simulink model "cpu_von_nuemann"  (R2020a)
settings: Solver=VariableStepAuto  StartTime=0.0  StopTime=10.0  RelTol=1e-3
libraries: simulink_extras x402, msbPllFoundation x1
(part 3 of 64)

== system cpu_von_nuemann/CPU/ALU/Multiplier/Subsystem3 ==
  In1 : Inport
  In2 : Inport  Port=2
  Constant17 : Constant  Value=0
  Demux : Demux  Outputs=16
  Demux1 : Demux  Outputs=16
  Display1 : Display
  Logical Operator : Logic  Operator=XOR  AllPortsSameDT=off  OutDataTypeStr=boolean
  Logical Operator1 : Logic  AllPortsSameDT=off  OutDataTypeStr=boolean
  Mux : Mux  Inputs=16
  Mux1 : Mux  Inputs=16
  Subsystem : Subsystem
  Subsystem1 : Subsystem
  Subsystem2 : Subsystem
  Subsystem3 : Subsystem
  Subsystem4 : Subsystem
  Subsystem5 : Subsystem
  Subsystem6 : Subsystem
  Out1 : Outport
  Out2 : Outport  Port=2
  wires:
  Subsystem3/11(Out11) -> Subsystem/27(In27)
  Subsystem5/16(Out16) -> Mux1/7
  Subsystem/16(Out16) -> Subsystem5/15(In23)
  Subsystem5/7(Out7) -> Subsystem6/30(In30)
  Subsystem2/14(Out14) -> Subsystem/14(In22)
  Subsystem4/9(Out9) -> Mux1/9
  Subsystem5/11(Out11) -> Mux1/2
  Subsystem2/15(Out15) -> Subsystem/15(In23)
  Subsystem3/16(Out16) -> Subsystem/32(In32)
  Subsystem3/6(Out6) -> Subsystem/22(In14)
  Subsystem6/10(Out10) -> Mux/9
  Subsystem5/2(Out2) -> Subsystem6/25(In25)
  Subsystem4/7(Out7) -> Subsystem5/31(In31)
  Subsystem2/11(Out11) -> Subsystem/11(In19)
  Subsystem3/9(Out9) -> Subsystem/25(In25)
  Subsystem1/2(Out2) -> Subsystem6/2(In2)
  Subsystem1/3(Out3) -> Subsystem6/3(In3)
  Subsystem/17(Out17) -> Subsystem5/16(In24)
  Subsystem/4(Out4) -> Subsystem5/3(In3)
  Subsystem3/8(Out8) -> Subsystem/24(In16)
  Subsystem/11(Out11) -> Subsystem5/10(In18)
  Logical Operator1/1 -> Subsystem6/23(In15)
  Subsystem3/2(Out2) -> Subsystem/18(In10)
  Subsystem1/13(Out13) -> Subsystem6/13(14)
  Subsystem4/4(Out4) -> Subsystem5/28(In28)
  Subsystem5/17(Out17) -> Mux1/8
  Subsystem5/5(Out5) -> Subsystem6/28(In28)
  Subsystem1/8(Out8) -> Subsystem6/8(In8)
  Subsystem2/3(Out3) -> Subsystem/3(In3)
  Subsystem5/6(Out6) -> Subsystem6/29(In29)
  Subsystem/2(Out2) -> Subsystem5/1(In1)
  Subsystem4/1(Out1) -> Subsystem5/25(In25)
  Subsystem1/7(Out7) -> Subsystem6/7(In7)
  Subsystem5/9(Out9) -> Subsystem6/32(In32)
  Subsystem6/8(Out8) -> Mux/7
  Subsystem1/5(Out5) -> Subsystem6/5(In5)
  Subsystem6/11(Out11) -> Mux/10
  Subsystem1/6(Out6) -> Subsystem6/6(In6)
  Subsystem/7(Out7) -> Subsystem5/6(In6)
  Subsystem2/16(Out16) -> Subsystem/16(In24)
  Demux/7 -> Subsystem2/7(In7), Subsystem1/7(In7)
  Demux1/14 -> Subsystem4/14(In14), Subsystem2/14(In14)
  Demux/16 -> Subsystem4/8(In8), Subsystem3/8(In8)
  Subsystem2/1(Out1) -> Subsystem/1(In1)
  Subsystem5/15(Out15) -> Mux1/6
  Subsystem4/16(Out16) -> Mux1/16
  Subsystem3/4(Out4) -> Subsystem/20(In12)
  Subsystem/1(Out1) -> Logical Operator1/2, Logical Operator/2
  Subsystem1/4(Out4) -> Subsystem6/4(In4)
  Subsystem4/11(Out11) -> Mux1/11
  Demux/1 -> Subsystem1/1(In1), Subsystem2/1(In1)
  Subsystem3/10(Out10) -> Subsystem/26(In26)
  Subsystem6/2(Out2) -> Mux/1
  Subsystem/9(Out9) -> Subsystem5/8(In8)
  Demux1/3 -> Subsystem3/11(In11), Subsystem1/11(In11)
  Demux1/7 -> Subsystem3/15(In15), Subsystem1/15(In15)
  Subsystem/5(Out5) -> Subsystem5/4(In4)
  Mux/1 -> Out1/1
  Subsystem5/10(Out10) -> Mux1/1
  Subsystem1/12(Out12) -> Subsystem6/12(In20)
  Subsystem2/6(Out6) -> Subsystem/6(In6)
  Demux/13 -> Subsystem4/5(In5), Subsystem3/5(In5)
  Demux/10 -> Subsystem4/2(In2), Subsystem3/2(In2)
  Demux/11 -> Subsystem4/3(In3), Subsystem3/3(In3)
  Subsystem1/11(Out11) -> Subsystem6/11(In19)
  Subsystem6/17(Out17) -> Mux/16
  Demux/9 -> Subsystem4/1(In1), Subsystem3/1(In1)
  Subsystem4/15(Out15) -> Mux1/15
  Subsystem5/8(Out8) -> Subsystem6/31(In31)
  Demux1/1 -> Subsystem1/9(In9), Subsystem3/9(In9)
  Demux1/2 -> Subsystem3/10(In10), Subsystem1/10(In10)
  Demux/8 -> Subsystem2/8(In8), Subsystem1/8(In8)
  Demux/14 -> Subsystem4/6(In6), Subsystem3/6(In6)
  Subsystem1/15(Out15) -> Subsystem6/15(In23)
  Demux1/9 -> Subsystem2/9(In9), Subsystem4/9(In9)
  Subsystem5/14(Out14) -> Mux1/5
  Demux/6 -> Subsystem1/6(In6), Subsystem2/6(In6)
  Subsystem2/7(Out7) -> Subsystem/7(In7)
  Subsystem2/4(Out4) -> Subsystem/4(In4)
  Demux1/5 -> Subsystem3/13(In13), Subsystem1/13(In13)
  Subsystem/8(Out8) -> Subsystem5/7(In7)
  Logical Operator/1 -> Subsystem6/24(In16)
  Demux1/12 -> Subsystem2/12(In12), Subsystem4/12(In12)
  Subsystem2/9(Out9) -> Subsystem/9(In17)
  Subsystem5/13(Out13) -> Mux1/4
  Subsystem5/3(Out3) -> Subsystem6/26(In26)
  Demux1/8 -> Subsystem1/16(In16), Subsystem3/16(In16)
  Subsystem4/14(Out14) -> Mux1/14
  Constant17/1 -> Subsystem5/24(In16), Subsystem5/23(In15), Subsystem5/22(In14), Subsystem5/21(In13), Subsystem5/20(In12), Subsystem5/19(In11), Subsystem5/18(In10), Subsystem5/17(In9), Subsystem6/17(In9), Subsystem6/18(In10), Subsystem6/20(In12), Subsystem6/21(In13), Subsystem6/22(In14), Subsystem6/19(In11)
  Subsystem3/13(Out13) -> Subsystem/29(In29)
  Subsystem1/16(Out16) -> Subsystem6/16(In24)
  Subsystem/15(Out15) -> Subsystem5/14(In22)
  Demux1/13 -> Subsystem2/13(In13), Subsystem4/13(In13)
  Subsystem/12(Out12) -> Subsystem5/11(In19)
  Demux1/16 -> Subsystem2/16(In16), Subsystem4/16(In16)
  Subsystem5/12(Out12) -> Mux1/3
  Subsystem3/15(Out15) -> Subsystem/31(In31)
  Subsystem6/9(Out9) -> Mux/8
  Demux/5 -> Subsystem1/5(In5), Subsystem2/5(In5)
  Subsystem6/4(Out4) -> Mux/3
  Subsystem6/3(Out3) -> Mux/2
  Subsystem4/13(Out13) -> Mux1/13
  Demux1/6 -> Subsystem3/14(In14), Subsystem1/14(In14)
  Subsystem/6(Out6) -> Subsystem5/5(In5)
  Subsystem/13(Out13) -> Subsystem5/12(In20)
  Subsystem6/13(Out13) -> Mux/12
  Subsystem6/12(Out12) -> Mux/11
  Subsystem4/10(Out10) -> Mux1/10
  Subsystem3/5(Out5) -> Subsystem/21(In13)
  Subsystem/10(Out10) -> Subsystem5/9(In17)
  Subsystem2/12(Out12) -> Subsystem/12(In20)
  Subsystem5/1(Out1) -> Logical Operator/1, Logical Operator1/1
  Subsystem6/5(Out5) -> Mux/4
  Subsystem3/1(Out1) -> Subsystem/17(In9)
  Subsystem4/8(Out8) -> Subsystem5/32(In32)
  Subsystem3/12(Out12) -> Subsystem/28(In28)
  Subsystem6/1(Out1) -> Display1/1
  Subsystem4/6(Out6) -> Subsystem5/30(In30)
  Subsystem2/2(Out2) -> Subsystem/2(In2)
  Subsystem2/10(Out10) -> Subsystem/10(In18)
  Subsystem4/5(Out5) -> Subsystem5/29(In29)
  Subsystem2/13(Out13) -> Subsystem/13(14)
  Subsystem1/1(Out1) -> Subsystem6/1(In1)
  Subsystem6/7(Out7) -> Mux/6
  Subsystem6/14(Out14) -> Mux/13
  Subsystem5/4(Out4) -> Subsystem6/27(In27)
  Subsystem2/8(Out8) -> Subsystem/8(In8)
  Subsystem/14(Out14) -> Subsystem5/13(14)
  Subsystem6/16(Out16) -> Mux/15
  Demux/4 -> Subsystem2/4(In4), Subsystem1/4(In4)
  Subsystem1/10(Out10) -> Subsystem6/10(In18)
  Demux/12 -> Subsystem4/4(In4), Subsystem3/4(In4)
  Subsystem3/14(Out14) -> Subsystem/30(In30)
  Subsystem2/5(Out5) -> Subsystem/5(In5)
  Demux1/10 -> Subsystem2/10(In10), Subsystem4/10(In10)
  Demux/2 -> Subsystem1/2(In2), Subsystem2/2(In2)
  Subsystem6/6(Out6) -> Mux/5
  Subsystem/3(Out3) -> Subsystem5/2(In2)
  Subsystem4/12(Out12) -> Mux1/12
  Demux1/4 -> Subsystem1/12(In12), Subsystem3/12(In12)
  Demux/15 -> Subsystem4/7(In7), Subsystem3/7(In7)
  Subsystem1/14(Out14) -> Subsystem6/14(In22)
  Subsystem3/3(Out3) -> Subsystem/19(In11)
  Subsystem6/15(Out15) -> Mux/14
  Subsystem1/9(Out9) -> Subsystem6/9(In17)
  Demux1/11 -> Subsystem2/11(In11), Subsystem4/11(In11)
  Subsystem4/2(Out2) -> Subsystem5/26(In26)
  Demux/3 -> Subsystem1/3(In3), Subsystem2/3(In3)
  Subsystem4/3(Out3) -> Subsystem5/27(In27)
  Subsystem3/7(Out7) -> Subsystem/23(In15)
  Demux1/15 -> Subsystem2/15(In15), Subsystem4/15(In15)
  In1/1 -> Demux/1
  In2/1 -> Demux1/1
  Mux1/1 -> Out2/1

== system cpu_von_nuemann/CPU/ALU/Multiplier/Subsystem4 ==
  In1 : Inport
  In2 : Inport  Port=2
  In3 : Inport  Port=3
  Demux : Demux  Outputs=2
  Demux1 : Demux  Outputs=2
  Mux : Mux  Inputs=2
  Subsystem1 : Subsystem
  Subsystem2 : Subsystem
  Out1 : Outport
  Out2 : Outport  Port=2
  wires:
  Mux/1 -> Out2/1
  In3/1 -> Demux1/1
  Subsystem2/2(Out2) -> Mux/2
  In1/1 -> Demux/1
  Subsystem2/1(Out1) -> Subsystem1/2(In2)
  Subsystem1/2(Out2) -> Mux/1
  Demux1/2 -> Subsystem2/3(In3)
  In2/1 -> Subsystem2/2(In2)
  Demux/2 -> Subsystem2/1(In1)
  Subsystem1/1(Out1) -> Out1/1
  Demux1/1 -> Subsystem1/3(In3)
  Demux/1 -> Subsystem1/1(In1)

== system cpu_von_nuemann/CPU/ALU/Multiplier/Subsystem5 ==
  In1 : Inport
  In2 : Inport  Port=2
  In3 : Inport  Port=3
  Demux : Demux  Outputs=2
  Demux1 : Demux  Outputs=2
  Mux : Mux  Inputs=2
  Subsystem : Subsystem
  Subsystem1 : Subsystem
  Out1 : Outport
  Out2 : Outport  Port=2
  wires:
  Mux/1 -> Out2/1
  Subsystem1/2(Out2) -> Mux/1
  In2/1 -> Subsystem/2(In2)
  Subsystem1/1(Out1) -> Out1/1
  Demux/2 -> Subsystem/1(In1)
  In3/1 -> Demux1/1
  Demux1/2 -> Subsystem/3(In3)
  Demux/1 -> Subsystem1/1(In1)
  Demux1/1 -> Subsystem1/3(In3)
  In1/1 -> Demux/1
  Subsystem/2(Out2) -> Mux/2
  Subsystem/1(Out1) -> Subsystem1/2(In2)

== system cpu_von_nuemann/CPU/ALU/Multiplier/Subsystem7 ==
  In1 : Inport
  In2 : Inport  Port=2
  Constant17 : Constant  Value=0
  Demux : Demux  Outputs=16
  Demux1 : Demux  Outputs=16
  Display1 : Display
  Logical Operator : Logic  Operator=XOR  AllPortsSameDT=off  OutDataTypeStr=boolean
  Logical Operator1 : Logic  AllPortsSameDT=off  OutDataTypeStr=boolean
  Mux : Mux  Inputs=16
  Mux1 : Mux  Inputs=16
  Subsystem : Subsystem
  Subsystem1 : Subsystem
  Subsystem2 : Subsystem
  Subsystem3 : Subsystem
  Subsystem4 : Subsystem
  Subsystem5 : Subsystem
  Subsystem6 : Subsystem
  Out1 : Outport
  Out2 : Outport  Port=2
  wires:
  Subsystem3/11(Out11) -> Subsystem/27(In27)
  Subsystem5/16(Out16) -> Mux1/7
  Subsystem/16(Out16) -> Subsystem5/15(In23)
  Subsystem5/7(Out7) -> Subsystem6/30(In30)
  Subsystem2/14(Out14) -> Subsystem/14(In22)
  Subsystem4/9(Out9) -> Mux1/9
  Subsystem5/11(Out11) -> Mux1/2
  Subsystem2/15(Out15) -> Subsystem/15(In23)
  Subsystem3/16(Out16) -> Subsystem/32(In32)
  Subsystem3/6(Out6) -> Subsystem/22(In14)
  Subsystem6/10(Out10) -> Mux/9
  Subsystem5/2(Out2) -> Subsystem6/25(In25)
  Subsystem4/7(Out7) -> Subsystem5/31(In31)
  Subsystem2/11(Out11) -> Subsystem/11(In19)
  Subsystem3/9(Out9) -> Subsystem/25(In25)
  Subsystem1/2(Out2) -> Subsystem6/2(In2)
  Subsystem1/3(Out3) -> Subsystem6/3(In3)
  Subsystem/17(Out17) -> Subsystem5/16(In24)
  Subsystem/4(Out4) -> Subsystem5/3(In3)
  Subsystem3/8(Out8) -> Subsystem/24(In16)
  Subsystem/11(Out11) -> Subsystem5/10(In18)
  Logical Operator1/1 -> Subsystem6/23(In15)
  Subsystem3/2(Out2) -> Subsystem/18(In10)
  Subsystem1/13(Out13) -> Subsystem6/13(14)
  Subsystem4/4(Out4) -> Subsystem5/28(In28)
  Subsystem5/17(Out17) -> Mux1/8
  Subsystem5/5(Out5) -> Subsystem6/28(In28)
  Subsystem1/8(Out8) -> Subsystem6/8(In8)
  Subsystem2/3(Out3) -> Subsystem/3(In3)
  Subsystem5/6(Out6) -> Subsystem6/29(In29)
  Subsystem/2(Out2) -> Subsystem5/1(In1)
  Subsystem4/1(Out1) -> Subsystem5/25(In25)
  Subsystem1/7(Out7) -> Subsystem6/7(In7)
  Subsystem5/9(Out9) -> Subsystem6/32(In32)
  Subsystem6/8(Out8) -> Mux/7
  Subsystem1/5(Out5) -> Subsystem6/5(In5)
  Subsystem6/11(Out11) -> Mux/10
  Subsystem1/6(Out6) -> Subsystem6/6(In6)
  Subsystem/7(Out7) -> Subsystem5/6(In6)
  Subsystem2/16(Out16) -> Subsystem/16(In24)
  Demux/7 -> Subsystem2/7(In7), Subsystem1/7(In7)
  Demux1/14 -> Subsystem4/14(In14), Subsystem2/14(In14)
  Demux/16 -> Subsystem4/8(In8), Subsystem3/8(In8)
  Subsystem2/1(Out1) -> Subsystem/1(In1)
  Subsystem5/15(Out15) -> Mux1/6
  Subsystem4/16(Out16) -> Mux1/16
  Subsystem3/4(Out4) -> Subsystem/20(In12)
  Subsystem/1(Out1) -> Logical Operator1/2, Logical Operator/2
  Subsystem1/4(Out4) -> Subsystem6/4(In4)
  Subsystem4/11(Out11) -> Mux1/11
  Demux/1 -> Subsystem1/1(In1), Subsystem2/1(In1)
  Subsystem3/10(Out10) -> Subsystem/26(In26)
  Subsystem6/2(Out2) -> Mux/1
  Subsystem/9(Out9) -> Subsystem5/8(In8)
  Demux1/3 -> Subsystem3/11(In11), Subsystem1/11(In11)
  Demux1/7 -> Subsystem3/15(In15), Subsystem1/15(In15)
  Subsystem/5(Out5) -> Subsystem5/4(In4)
  Mux/1 -> Out1/1
  Subsystem5/10(Out10) -> Mux1/1
  Subsystem1/12(Out12) -> Subsystem6/12(In20)
  Subsystem2/6(Out6) -> Subsystem/6(In6)
  Demux/13 -> Subsystem4/5(In5), Subsystem3/5(In5)
  Demux/10 -> Subsystem4/2(In2), Subsystem3/2(In2)
  Demux/11 -> Subsystem4/3(In3), Subsystem3/3(In3)
  Subsystem1/11(Out11) -> Subsystem6/11(In19)
  Subsystem6/17(Out17) -> Mux/16
  Demux/9 -> Subsystem4/1(In1), Subsystem3/1(In1)
  Subsystem4/15(Out15) -> Mux1/15
  Subsystem5/8(Out8) -> Subsystem6/31(In31)
  Demux1/1 -> Subsystem1/9(In9), Subsystem3/9(In9)
  Demux1/2 -> Subsystem3/10(In10), Subsystem1/10(In10)
  Demux/8 -> Subsystem2/8(In8), Subsystem1/8(In8)
  Demux/14 -> Subsystem4/6(In6), Subsystem3/6(In6)
  Subsystem1/15(Out15) -> Subsystem6/15(In23)
  Demux1/9 -> Subsystem2/9(In9), Subsystem4/9(In9)
  Subsystem5/14(Out14) -> Mux1/5
  Demux/6 -> Subsystem1/6(In6), Subsystem2/6(In6)
  Subsystem2/7(Out7) -> Subsystem/7(In7)
  Subsystem2/4(Out4) -> Subsystem/4(In4)
  Demux1/5 -> Subsystem3/13(In13), Subsystem1/13(In13)
  Subsystem/8(Out8) -> Subsystem5/7(In7)
  Logical Operator/1 -> Subsystem6/24(In16)
  Demux1/12 -> Subsystem2/12(In12), Subsystem4/12(In12)
  Subsystem2/9(Out9) -> Subsystem/9(In17)
  Subsystem5/13(Out13) -> Mux1/4
  Subsystem5/3(Out3) -> Subsystem6/26(In26)
  Demux1/8 -> Subsystem1/16(In16), Subsystem3/16(In16)
  Subsystem4/14(Out14) -> Mux1/14
  Constant17/1 -> Subsystem5/24(In16), Subsystem5/23(In15), Subsystem5/22(In14), Subsystem5/21(In13), Subsystem5/20(In12), Subsystem5/19(In11), Subsystem5/18(In10), Subsystem5/17(In9), Subsystem6/17(In9), Subsystem6/18(In10), Subsystem6/20(In12), Subsystem6/21(In13), Subsystem6/22(In14), Subsystem6/19(In11)
  Subsystem3/13(Out13) -> Subsystem/29(In29)
  Subsystem1/16(Out16) -> Subsystem6/16(In24)
  Subsystem/15(Out15) -> Subsystem5/14(In22)
  Demux1/13 -> Subsystem2/13(In13), Subsystem4/13(In13)
  Subsystem/12(Out12) -> Subsystem5/11(In19)
  Demux1/16 -> Subsystem2/16(In16), Subsystem4/16(In16)
  Subsystem5/12(Out12) -> Mux1/3
  Subsystem3/15(Out15) -> Subsystem/31(In31)
  Subsystem6/9(Out9) -> Mux/8
  Demux/5 -> Subsystem1/5(In5), Subsystem2/5(In5)
  Subsystem6/4(Out4) -> Mux/3
  Subsystem6/3(Out3) -> Mux/2
  Subsystem4/13(Out13) -> Mux1/13
  Demux1/6 -> Subsystem3/14(In14), Subsystem1/14(In14)
  Subsystem/6(Out6) -> Subsystem5/5(In5)
  Subsystem/13(Out13) -> Subsystem5/12(In20)
  Subsystem6/13(Out13) -> Mux/12
  Subsystem6/12(Out12) -> Mux/11
  Subsystem4/10(Out10) -> Mux1/10
  Subsystem3/5(Out5) -> Subsystem/21(In13)
  Subsystem/10(Out10) -> Subsystem5/9(In17)
  Subsystem2/12(Out12) -> Subsystem/12(In20)
  Subsystem5/1(Out1) -> Logical Operator/1, Logical Operator1/1
  Subsystem6/5(Out5) -> Mux/4
  Subsystem3/1(Out1) -> Subsystem/17(In9)
  Subsystem4/8(Out8) -> Subsystem5/32(In32)
  Subsystem3/12(Out12) -> Subsystem/28(In28)
  Subsystem6/1(Out1) -> Display1/1
  Subsystem4/6(Out6) -> Subsystem5/30(In30)
  Subsystem2/2(Out2) -> Subsystem/2(In2)
  Subsystem2/10(Out10) -> Subsystem/10(In18)
  Subsystem4/5(Out5) -> Subsystem5/29(In29)
  Subsystem2/13(Out13) -> Subsystem/13(14)
  Subsystem1/1(Out1) -> Subsystem6/1(In1)
  Subsystem6/7(Out7) -> Mux/6
  Subsystem6/14(Out14) -> Mux/13
  Subsystem5/4(Out4) -> Subsystem6/27(In27)
  Subsystem2/8(Out8) -> Subsystem/8(In8)
  Subsystem/14(Out14) -> Subsystem5/13(14)
  Subsystem6/16(Out16) -> Mux/15
  Demux/4 -> Subsystem2/4(In4), Subsystem1/4(In4)
  Subsystem1/10(Out10) -> Subsystem6/10(In18)
  Demux/12 -> Subsystem4/4(In4), Subsystem3/4(In4)
  Subsystem3/14(Out14) -> Subsystem/30(In30)
  Subsystem2/5(Out5) -> Subsystem/5(In5)
  Demux1/10 -> Subsystem2/10(In10), Subsystem4/10(In10)
  Demux/2 -> Subsystem1/2(In2), Subsystem2/2(In2)
  Subsystem6/6(Out6) -> Mux/5
  Subsystem/3(Out3) -> Subsystem5/2(In2)
  Subsystem4/12(Out12) -> Mux1/12
  Demux1/4 -> Subsystem1/12(In12), Subsystem3/12(In12)
  Demux/15 -> Subsystem4/7(In7), Subsystem3/7(In7)
  Subsystem1/14(Out14) -> Subsystem6/14(In22)
  Subsystem3/3(Out3) -> Subsystem/19(In11)
  Subsystem6/15(Out15) -> Mux/14
  Subsystem1/9(Out9) -> Subsystem6/9(In17)
  Demux1/11 -> Subsystem2/11(In11), Subsystem4/11(In11)
  Subsystem4/2(Out2) -> Subsystem5/26(In26)
  Demux/3 -> Subsystem1/3(In3), Subsystem2/3(In3)
  Subsystem4/3(Out3) -> Subsystem5/27(In27)
  Subsystem3/7(Out7) -> Subsystem/23(In15)
  Demux1/15 -> Subsystem2/15(In15), Subsystem4/15(In15)
  In1/1 -> Demux/1
  In2/1 -> Demux1/1
  Mux1/1 -> Out2/1

== system cpu_von_nuemann/CPU/ALU/Subsystem7/Subsystem1 ==
  In20 : Inport
  In21 : Inport  Port=2
  In1 : Inport  Port=3
  In2 : Inport  Port=4
  In3 : Inport  Port=5
  In4 : Inport  Port=6
  In5 : Inport  Port=7
  In6 : Inport  Port=8
  In7 : Inport  Port=9
  In8 : Inport  Port=10
  In9 : Inport  Port=11
  In10 : Inport  Port=12
  In11 : Inport  Port=13
  In12 : Inport  Port=14
  In13 : Inport  Port=15
  In14 : Inport  Port=16
  In15 : Inport  Port=17
  In16 : Inport  Port=18
  In17 : Inport  Port=19
  In18 : Inport  Port=20
  In19 : Inport  Port=21
  Subsystem1 : Subsystem
  Subsystem2 : Subsystem
  Subsystem3 : Subsystem
  Subsystem4 : Subsystem
  Subsystem5 : Subsystem
  Out1 : Outport
  wires:
  Subsystem4/1(Out1) -> Subsystem5/3(In3)
  Subsystem1/1(Out1) -> Subsystem5/4(In4)
  Subsystem2/1(Out1) -> Subsystem5/5(In5)
  Subsystem3/1(Out1) -> Subsystem5/6(In7)
  Subsystem5/1(Out1) -> Out1/1
  In1/1 -> Subsystem4/1(In1), Subsystem1/1(In1), Subsystem3/1(In1), Subsystem2/1(In1)
  In2/1 -> Subsystem4/2(In2), Subsystem1/2(In2), Subsystem3/2(In2), Subsystem2/2(In2)
  In19/1 -> Subsystem5/7(In6), Subsystem3/7(In6), Subsystem2/7(In6), Subsystem1/7(In6), Subsystem4/7(In6)
  In3/1 -> Subsystem4/3(In3)
  In4/1 -> Subsystem4/4(In4)
  In6/1 -> Subsystem4/6(In7)
  In5/1 -> Subsystem4/5(In5)
  In8/1 -> Subsystem1/4(In4)
  In9/1 -> Subsystem1/5(In5)
  In7/1 -> Subsystem1/3(In3)
  In10/1 -> Subsystem1/6(In7)
  In15/1 -> Subsystem3/3(In3)
  In18/1 -> Subsystem3/6(In7)
  In13/1 -> Subsystem2/5(In5)
  In12/1 -> Subsystem2/4(In4)
  In17/1 -> Subsystem3/5(In5)
  In16/1 -> Subsystem3/4(In4)
  In11/1 -> Subsystem2/3(In3)
  In14/1 -> Subsystem2/6(In7)
  In20/1 -> Subsystem5/1(In1)
  In21/1 -> Subsystem5/2(In2)

== system cpu_von_nuemann/CPU/ALU/Subsystem7/Subsystem2 ==
  In20 : Inport
  In21 : Inport  Port=2
  In1 : Inport  Port=3
  In2 : Inport  Port=4
  In3 : Inport  Port=5
  In4 : Inport  Port=6
  In5 : Inport  Port=7
  In6 : Inport  Port=8
  In7 : Inport  Port=9
  In8 : Inport  Port=10
  In9 : Inport  Port=11
  In10 : Inport  Port=12
  In11 : Inport  Port=13
  In12 : Inport  Port=14
  In13 : Inport  Port=15
  In14 : Inport  Port=16
  In15 : Inport  Port=17
  In16 : Inport  Port=18
  In17 : Inport  Port=19
  In18 : Inport  Port=20
  In19 : Inport  Port=21
  Subsystem1 : Subsystem
  Subsystem2 : Subsystem
  Subsystem3 : Subsystem
  Subsystem4 : Subsystem
  Subsystem5 : Subsystem
  Out1 : Outport
  wires:
  Subsystem4/1(Out1) -> Subsystem5/3(In3)
  Subsystem1/1(Out1) -> Subsystem5/4(In4)
  Subsystem2/1(Out1) -> Subsystem5/5(In5)
  Subsystem3/1(Out1) -> Subsystem5/6(In7)
  Subsystem5/1(Out1) -> Out1/1
  In1/1 -> Subsystem4/1(In1), Subsystem1/1(In1), Subsystem3/1(In1), Subsystem2/1(In1)
  In2/1 -> Subsystem4/2(In2), Subsystem1/2(In2), Subsystem3/2(In2), Subsystem2/2(In2)
  In19/1 -> Subsystem5/7(In6), Subsystem3/7(In6), Subsystem2/7(In6), Subsystem1/7(In6), Subsystem4/7(In6)
  In3/1 -> Subsystem4/3(In3)
  In4/1 -> Subsystem4/4(In4)
  In6/1 -> Subsystem4/6(In7)
  In5/1 -> Subsystem4/5(In5)
  In8/1 -> Subsystem1/4(In4)
  In9/1 -> Subsystem1/5(In5)
  In7/1 -> Subsystem1/3(In3)
  In10/1 -> Subsystem1/6(In7)
  In15/1 -> Subsystem3/3(In3)
  In18/1 -> Subsystem3/6(In7)
  In13/1 -> Subsystem2/5(In5)
  In12/1 -> Subsystem2/4(In4)
  In17/1 -> Subsystem3/5(In5)
  In16/1 -> Subsystem3/4(In4)
  In11/1 -> Subsystem2/3(In3)
  In14/1 -> Subsystem2/6(In7)
  In20/1 -> Subsystem5/1(In1)
  In21/1 -> Subsystem5/2(In2)

== system cpu_von_nuemann/CPU/ALU/Subsystem7/Subsystem3 ==
  In20 : Inport
  In21 : Inport  Port=2
  In1 : Inport  Port=3
  In2 : Inport  Port=4
  In3 : Inport  Port=5
  In4 : Inport  Port=6
  In5 : Inport  Port=7
  In6 : Inport  Port=8
  In7 : Inport  Port=9
  In8 : Inport  Port=10
  In9 : Inport  Port=11
  In10 : Inport  Port=12
  In11 : Inport  Port=13
  In12 : Inport  Port=14
  In13 : Inport  Port=15
  In14 : Inport  Port=16
  In15 : Inport  Port=17
  In16 : Inport  Port=18
  In17 : Inport  Port=19
  In18 : Inport  Port=20
  In19 : Inport  Port=21
  Subsystem1 : Subsystem
  Subsystem2 : Subsystem
  Subsystem3 : Subsystem
  Subsystem4 : Subsystem
  Subsystem5 : Subsystem
  Out1 : Outport
  wires:
  Subsystem4/1(Out1) -> Subsystem5/3(In3)
  Subsystem1/1(Out1) -> Subsystem5/4(In4)
  Subsystem2/1(Out1) -> Subsystem5/5(In5)
  Subsystem3/1(Out1) -> Subsystem5/6(In7)
  Subsystem5/1(Out1) -> Out1/1
  In1/1 -> Subsystem4/1(In1), Subsystem1/1(In1), Subsystem3/1(In1), Subsystem2/1(In1)
  In2/1 -> Subsystem4/2(In2), Subsystem1/2(In2), Subsystem3/2(In2), Subsystem2/2(In2)
  In19/1 -> Subsystem5/7(In6), Subsystem3/7(In6), Subsystem2/7(In6), Subsystem1/7(In6), Subsystem4/7(In6)
  In3/1 -> Subsystem4/3(In3)
  In4/1 -> Subsystem4/4(In4)
  In6/1 -> Subsystem4/6(In7)
  In5/1 -> Subsystem4/5(In5)
  In8/1 -> Subsystem1/4(In4)
  In9/1 -> Subsystem1/5(In5)
  In7/1 -> Subsystem1/3(In3)
  In10/1 -> Subsystem1/6(In7)
  In15/1 -> Subsystem3/3(In3)
  In18/1 -> Subsystem3/6(In7)
  In13/1 -> Subsystem2/5(In5)
  In12/1 -> Subsystem2/4(In4)
  In17/1 -> Subsystem3/5(In5)
  In16/1 -> Subsystem3/4(In4)
  In11/1 -> Subsystem2/3(In3)
  In14/1 -> Subsystem2/6(In7)
  In20/1 -> Subsystem5/1(In1)
  In21/1 -> Subsystem5/2(In2)

== system cpu_von_nuemann/CPU/ALU/Subsystem7/Subsystem4 ==
  In20 : Inport
  In21 : Inport  Port=2
  In1 : Inport  Port=3
  In2 : Inport  Port=4
  In3 : Inport  Port=5
  In4 : Inport  Port=6
  In5 : Inport  Port=7
  In6 : Inport  Port=8
  In7 : Inport  Port=9
  In8 : Inport  Port=10
  In9 : Inport  Port=11
  In10 : Inport  Port=12
  In11 : Inport  Port=13
  In12 : Inport  Port=14
  In13 : Inport  Port=15
  In14 : Inport  Port=16
  In15 : Inport  Port=17
  In16 : Inport  Port=18
  In17 : Inport  Port=19
  In18 : Inport  Port=20
  In19 : Inport  Port=21
  Subsystem1 : Subsystem
  Subsystem2 : Subsystem
  Subsystem3 : Subsystem
  Subsystem4 : Subsystem
  Subsystem5 : Subsystem
  Out1 : Outport
  wires:
  Subsystem4/1(Out1) -> Subsystem5/3(In3)
  Subsystem1/1(Out1) -> Subsystem5/4(In4)
  Subsystem2/1(Out1) -> Subsystem5/5(In5)
  Subsystem3/1(Out1) -> Subsystem5/6(In7)
  Subsystem5/1(Out1) -> Out1/1
  In1/1 -> Subsystem4/1(In1), Subsystem1/1(In1), Subsystem3/1(In1), Subsystem2/1(In1)
  In2/1 -> Subsystem4/2(In2), Subsystem1/2(In2), Subsystem3/2(In2), Subsystem2/2(In2)
  In19/1 -> Subsystem5/7(In6), Subsystem3/7(In6), Subsystem2/7(In6), Subsystem1/7(In6), Subsystem4/7(In6)
  In3/1 -> Subsystem4/3(In3)
  In4/1 -> Subsystem4/4(In4)
  In6/1 -> Subsystem4/6(In7)
  In5/1 -> Subsystem4/5(In5)
  In8/1 -> Subsystem1/4(In4)
  In9/1 -> Subsystem1/5(In5)
  In7/1 -> Subsystem1/3(In3)
  In10/1 -> Subsystem1/6(In7)
  In15/1 -> Subsystem3/3(In3)
  In18/1 -> Subsystem3/6(In7)
  In13/1 -> Subsystem2/5(In5)
  In12/1 -> Subsystem2/4(In4)
  In17/1 -> Subsystem3/5(In5)
  In16/1 -> Subsystem3/4(In4)
  In11/1 -> Subsystem2/3(In3)
  In14/1 -> Subsystem2/6(In7)
  In20/1 -> Subsystem5/1(In1)
  In21/1 -> Subsystem5/2(In2)

== system cpu_von_nuemann/CPU/ALU/Subtractor/Subtractor ==
  In1 : Inport
  In2 : Inport  Port=2
  In3 : Inport  Port=3
  Demux : Demux  Outputs=2
  Demux1 : Demux  Outputs=2
  Mux : Mux  Inputs=2
  Subsystem1 : Subsystem
  Subsystem2 : Subsystem
  Out1 : Outport
  Out2 : Outport  Port=2
  wires:
  Mux/1 -> Out2/1
  In3/1 -> Demux1/1
  Subsystem2/2(Out2) -> Mux/2
  In1/1 -> Demux/1
  Subsystem2/1(Out1) -> Subsystem1/2(In2)
  Subsystem1/2(Out2) -> Mux/1
  Demux1/2 -> Subsystem2/3(In3)
  In2/1 -> Subsystem2/2(In2)
  Demux/2 -> Subsystem2/1(In1)
  Subsystem1/1(Out1) -> Out1/1
  Demux1/1 -> Subsystem1/3(In3)
  Demux/1 -> Subsystem1/1(In1)

== system cpu_von_nuemann/CPU/CU/Subsystem4/Subsystem1 ==
  In1 : Inport
  In2 : Inport  Port=2
  In3 : Inport  Port=3
  In4 : Inport  Port=4
  In5 : Inport  Port=5
  Logical Operator{,1..15} (16 alike) : Logic  Inputs=5  AllPortsSameDT=off  OutDataTypeStr=boolean
  Logical Operator{16..19} (4 alike) : Logic  Operator=NOT  Inputs=5  AllPortsSameDT=off  OutDataTypeStr=boolean
  Out1 : Outport
  Out2 : Outport  Port=2
  Out3 : Outport  Port=3
  Out4 : Outport  Port=4
  Out5 : Outport  Port=5
  Out6 : Outport  Port=6
  Out7 : Outport  Port=7
  Out8 : Outport  Port=8
  Out9 : Outport  Port=9
  Out10 : Outport  Port=10
  Out11 : Outport  Port=11
  Out12 : Outport  Port=12
  Out13 : Outport  Port=13
  Out14 : Outport  Port=14
  Out15 : Outport  Port=15
  Out16 : Outport  Port=16
  wires:
  Logical Operator18/1 -> Logical Operator11/1, Logical Operator10/1, Logical Operator5/1, Logical Operator4/1, Logical Operator3/1, Logical Operator2/1, Logical Operator1/1, Logical Operator/1
  In4/1 -> Logical Operator9/4, Logical Operator15/4, Logical Operator13/4, Logical Operator7/4, Logical Operator11/4, Logical Operator5/4, Logical Operator3/4, Logical Operator1/4, Logical Operator19/1
  Logical Operator17/1 -> Logical Operator13/2, Logical Operator12/2, Logical Operator7/2, Logical Operator6/2, Logical Operator3/2, Logical Operator2/2, Logical Operator1/2, Logical Operator/2
  In2/1 -> Logical Operator4/2, Logical Operator5/2, Logical Operator10/2, Logical Operator14/2, Logical Operator15/2, Logical Operator8/2, Logical Operator9/2, Logical Operator11/2, Logical Operator17/1
  Logical Operator19/1 -> Logical Operator8/4, Logical Operator14/4, Logical Operator12/4, Logical Operator6/4, Logical Operator10/4, Logical Operator4/4, Logical Operator2/4, Logical Operator/4
  In5/1 -> Logical Operator9/5, Logical Operator8/5, Logical Operator15/5, Logical Operator14/5, Logical Operator13/5, Logical Operator12/5, Logical Operator7/5, Logical Operator6/5, Logical Operator11/5, Logical Operator10/5, Logical Operator5/5, Logical Operator4/5, Logical Operator3/5, Logical Operator2/5, Logical Operator1/5, Logical Operator/5
  Logical Operator16/1 -> Logical Operator15/3, Logical Operator14/3, Logical Operator7/3, Logical Operator6/3, Logical Operator5/3, Logical Operator4/3, Logical Operator1/3, Logical Operator/3
  In3/1 -> Logical Operator9/3, Logical Operator8/3, Logical Operator13/3, Logical Operator12/3, Logical Operator11/3, Logical Operator10/3, Logical Operator3/3, Logical Operator2/3, Logical Operator16/1
  In1/1 -> Logical Operator6/1, Logical Operator7/1, Logical Operator12/1, Logical Operator13/1, Logical Operator14/1, Logical Operator15/1, Logical Operator8/1, Logical Operator9/1, Logical Operator18/1
  Logical Operator/1 -> Out1/1
  Logical Operator1/1 -> Out2/1
  Logical Operator2/1 -> Out3/1
  Logical Operator3/1 -> Out4/1
  Logical Operator5/1 -> Out6/1
  Logical Operator4/1 -> Out5/1
  Logical Operator10/1 -> Out7/1
  Logical Operator11/1 -> Out8/1
  Logical Operator14/1 -> Out13/1
  Logical Operator15/1 -> Out14/1
  Logical Operator8/1 -> Out15/1
  Logical Operator7/1 -> Out10/1
  Logical Operator6/1 -> Out9/1
  Logical Operator12/1 -> Out11/1
  Logical Operator13/1 -> Out12/1
  Logical Operator9/1 -> Out16/1

== system cpu_von_nuemann/CPU/MU/Accumulator/Subsystem ==
  In1 : Inport
  In2 : Inport  Port=2
  In3 : Inport  Port=3
  D Flip-Flop{,1..7} (8 alike) : simulink_extras/Flip Flops/D Flip-Flop
  Demux : Demux  Outputs=8
  Display : Display
  Mux : Mux  Inputs=8
  Mux1 : Mux  Inputs=8
  Out1 : Outport
  wires:
  D Flip-Flop6/2 -> Mux1/7
  D Flip-Flop1/2 -> Mux1/2
  Demux/5 -> D Flip-Flop4/1
  D Flip-Flop1/1 -> Mux/2
  D Flip-Flop2/1 -> Mux/3
  D Flip-Flop5/1 -> Mux/6
  Demux/6 -> D Flip-Flop5/1
  In3/1 -> D Flip-Flop7/3, D Flip-Flop6/3, D Flip-Flop5/3, D Flip-Flop4/3, D Flip-Flop3/3, D Flip-Flop2/3, D Flip-Flop1/3, D Flip-Flop/3
  Demux/7 -> D Flip-Flop6/1
  D Flip-Flop6/1 -> Mux/7
  Demux/3 -> D Flip-Flop2/1
  Mux/1 -> Out1/1
  In2/1 -> D Flip-Flop7/2, D Flip-Flop6/2, D Flip-Flop5/2, D Flip-Flop4/2, D Flip-Flop3/2, D Flip-Flop2/2, D Flip-Flop/2, D Flip-Flop1/2
  Demux/2 -> D Flip-Flop1/1
  Demux/8 -> D Flip-Flop7/1
  D Flip-Flop5/2 -> Mux1/6
  D Flip-Flop4/1 -> Mux/5
  D Flip-Flop7/2 -> Mux1/8
  D Flip-Flop7/1 -> Mux/8
  Demux/4 -> D Flip-Flop3/1
  Mux1/1 -> Display/1
  D Flip-Flop2/2 -> Mux1/3
  In1/1 -> Demux/1
  D Flip-Flop4/2 -> Mux1/5
  Demux/1 -> D Flip-Flop/1
  D Flip-Flop/2 -> Mux1/1
  D Flip-Flop3/1 -> Mux/4
  D Flip-Flop/1 -> Mux/1
  D Flip-Flop3/2 -> Mux1/4

== system cpu_von_nuemann/CPU/MU/Accumulator/Subsystem1 ==
  In1 : Inport
  In2 : Inport  Port=2
  In3 : Inport  Port=3
  D Flip-Flop{,1..7} (8 alike) : simulink_extras/Flip Flops/D Flip-Flop
  Demux : Demux  Outputs=8
  Display : Display
  Mux : Mux  Inputs=8
  Mux1 : Mux  Inputs=8
  Out1 : Outport
  wires:
  D Flip-Flop6/2 -> Mux1/7
  D Flip-Flop1/2 -> Mux1/2
  Demux/5 -> D Flip-Flop4/1
  D Flip-Flop1/1 -> Mux/2
  D Flip-Flop2/1 -> Mux/3
  D Flip-Flop5/1 -> Mux/6
  Demux/6 -> D Flip-Flop5/1
  In3/1 -> D Flip-Flop7/3, D Flip-Flop6/3, D Flip-Flop5/3, D Flip-Flop4/3, D Flip-Flop3/3, D Flip-Flop2/3, D Flip-Flop1/3, D Flip-Flop/3
  Demux/7 -> D Flip-Flop6/1
  D Flip-Flop6/1 -> Mux/7
  Demux/3 -> D Flip-Flop2/1
  Mux/1 -> Out1/1
  In2/1 -> D Flip-Flop7/2, D Flip-Flop6/2, D Flip-Flop5/2, D Flip-Flop4/2, D Flip-Flop3/2, D Flip-Flop2/2, D Flip-Flop/2, D Flip-Flop1/2
  Demux/2 -> D Flip-Flop1/1
  Demux/8 -> D Flip-Flop7/1
  D Flip-Flop5/2 -> Mux1/6
  D Flip-Flop4/1 -> Mux/5
  D Flip-Flop7/2 -> Mux1/8
  D Flip-Flop7/1 -> Mux/8
  Demux/4 -> D Flip-Flop3/1
  Mux1/1 -> Display/1
  D Flip-Flop2/2 -> Mux1/3
  In1/1 -> Demux/1
  D Flip-Flop4/2 -> Mux1/5
  Demux/1 -> D Flip-Flop/1
  D Flip-Flop/2 -> Mux1/1
  D Flip-Flop3/1 -> Mux/4
  D Flip-Flop/1 -> Mux/1
  D Flip-Flop3/2 -> Mux1/4

== system cpu_von_nuemann/CPU/MU/Accumulator/Subsystem2 ==
  In1 : Inport
  In2 : Inport  Port=2
  In3 : Inport  Port=3
  D Flip-Flop{,1..7} (8 alike) : simulink_extras/Flip Flops/D Flip-Flop
  Demux : Demux  Outputs=8
  Display : Display
  Mux : Mux  Inputs=8
  Mux1 : Mux  Inputs=8
  Out1 : Outport
  wires:
  D Flip-Flop6/2 -> Mux1/7
  D Flip-Flop1/2 -> Mux1/2
  Demux/5 -> D Flip-Flop4/1
  D Flip-Flop1/1 -> Mux/2
  D Flip-Flop2/1 -> Mux/3
  D Flip-Flop5/1 -> Mux/6
  Demux/6 -> D Flip-Flop5/1
  In3/1 -> D Flip-Flop7/3, D Flip-Flop6/3, D Flip-Flop5/3, D Flip-Flop4/3, D Flip-Flop3/3, D Flip-Flop2/3, D Flip-Flop1/3, D Flip-Flop/3
  Demux/7 -> D Flip-Flop6/1
  D Flip-Flop6/1 -> Mux/7
  Demux/3 -> D Flip-Flop2/1
  Mux/1 -> Out1/1
  In2/1 -> D Flip-Flop7/2, D Flip-Flop6/2, D Flip-Flop5/2, D Flip-Flop4/2, D Flip-Flop3/2, D Flip-Flop2/2, D Flip-Flop/2, D Flip-Flop1/2
  Demux/2 -> D Flip-Flop1/1
  Demux/8 -> D Flip-Flop7/1
  D Flip-Flop5/2 -> Mux1/6
  D Flip-Flop4/1 -> Mux/5
  D Flip-Flop7/2 -> Mux1/8
  D Flip-Flop7/1 -> Mux/8
  Demux/4 -> D Flip-Flop3/1
  Mux1/1 -> Display/1
  D Flip-Flop2/2 -> Mux1/3
  In1/1 -> Demux/1
  D Flip-Flop4/2 -> Mux1/5
  Demux/1 -> D Flip-Flop/1
  D Flip-Flop/2 -> Mux1/1
  D Flip-Flop3/1 -> Mux/4
  D Flip-Flop/1 -> Mux/1
  D Flip-Flop3/2 -> Mux1/4

== system cpu_von_nuemann/CPU/MU/Accumulator/Subsystem3 ==
  In1 : Inport
  In2 : Inport  Port=2
  In3 : Inport  Port=3
  D Flip-Flop{,1..7} (8 alike) : simulink_extras/Flip Flops/D Flip-Flop
  Demux : Demux  Outputs=8
  Display : Display
  Mux : Mux  Inputs=8
  Mux1 : Mux  Inputs=8
  Out1 : Outport
  wires:
  D Flip-Flop6/2 -> Mux1/7
  D Flip-Flop1/2 -> Mux1/2
  Demux/5 -> D Flip-Flop4/1
  D Flip-Flop1/1 -> Mux/2
  D Flip-Flop2/1 -> Mux/3
  D Flip-Flop5/1 -> Mux/6
  Demux/6 -> D Flip-Flop5/1
  In3/1 -> D Flip-Flop7/3, D Flip-Flop6/3, D Flip-Flop5/3, D Flip-Flop4/3, D Flip-Flop3/3, D Flip-Flop2/3, D Flip-Flop1/3, D Flip-Flop/3
  Demux/7 -> D Flip-Flop6/1
  D Flip-Flop6/1 -> Mux/7
  Demux/3 -> D Flip-Flop2/1
  Mux/1 -> Out1/1
  In2/1 -> D Flip-Flop7/2, D Flip-Flop6/2, D Flip-Flop5/2, D Flip-Flop4/2, D Flip-Flop3/2, D Flip-Flop2/2, D Flip-Flop/2, D Flip-Flop1/2
  Demux/2 -> D Flip-Flop1/1
  Demux/8 -> D Flip-Flop7/1
  D Flip-Flop5/2 -> Mux1/6
  D Flip-Flop4/1 -> Mux/5
  D Flip-Flop7/2 -> Mux1/8
  D Flip-Flop7/1 -> Mux/8
  Demux/4 -> D Flip-Flop3/1
  Mux1/1 -> Display/1
  D Flip-Flop2/2 -> Mux1/3
  In1/1 -> Demux/1
  D Flip-Flop4/2 -> Mux1/5
  Demux/1 -> D Flip-Flop/1
  D Flip-Flop/2 -> Mux1/1
  D Flip-Flop3/1 -> Mux/4
  D Flip-Flop/1 -> Mux/1
  D Flip-Flop3/2 -> Mux1/4

== system cpu_von_nuemann/CPU/MU/Multiplier H bit/Subsystem ==
  In1 : Inport
  In2 : Inport  Port=2
  In3 : Inport  Port=3
  D Flip-Flop{,1..7} (8 alike) : simulink_extras/Flip Flops/D Flip-Flop
  Demux : Demux  Outputs=8
  Display : Display
  Mux : Mux  Inputs=8
  Mux1 : Mux  Inputs=8
  Out1 : Outport
  wires:
  D Flip-Flop6/2 -> Mux1/7
  D Flip-Flop1/2 -> Mux1/2
  Demux/5 -> D Flip-Flop4/1
  D Flip-Flop1/1 -> Mux/2
  D Flip-Flop2/1 -> Mux/3
  D Flip-Flop5/1 -> Mux/6
  Demux/6 -> D Flip-Flop5/1
  In3/1 -> D Flip-Flop7/3, D Flip-Flop6/3, D Flip-Flop5/3, D Flip-Flop4/3, D Flip-Flop3/3, D Flip-Flop2/3, D Flip-Flop1/3, D Flip-Flop/3
  Demux/7 -> D Flip-Flop6/1
  D Flip-Flop6/1 -> Mux/7
  Demux/3 -> D Flip-Flop2/1
  Mux/1 -> Out1/1
  In2/1 -> D Flip-Flop7/2, D Flip-Flop6/2, D Flip-Flop5/2, D Flip-Flop4/2, D Flip-Flop3/2, D Flip-Flop2/2, D Flip-Flop/2, D Flip-Flop1/2
  Demux/2 -> D Flip-Flop1/1
  Demux/8 -> D Flip-Flop7/1
  D Flip-Flop5/2 -> Mux1/6
  D Flip-Flop4/1 -> Mux/5
  D Flip-Flop7/2 -> Mux1/8
  D Flip-Flop7/1 -> Mux/8
  Demux/4 -> D Flip-Flop3/1
  Mux1/1 -> Display/1
  D Flip-Flop2/2 -> Mux1/3
  In1/1 -> Demux/1
  D Flip-Flop4/2 -> Mux1/5
  Demux/1 -> D Flip-Flop/1
  D Flip-Flop/2 -> Mux1/1
  D Flip-Flop3/1 -> Mux/4
  D Flip-Flop/1 -> Mux/1
  D Flip-Flop3/2 -> Mux1/4

== system cpu_von_nuemann/CPU/MU/Multiplier H bit/Subsystem1 ==
  In1 : Inport
  In2 : Inport  Port=2
  In3 : Inport  Port=3
  D Flip-Flop{,1..7} (8 alike) : simulink_extras/Flip Flops/D Flip-Flop
  Demux : Demux  Outputs=8
  Display : Display
  Mux : Mux  Inputs=8
  Mux1 : Mux  Inputs=8
  Out1 : Outport
  wires:
  D Flip-Flop6/2 -> Mux1/7
  D Flip-Flop1/2 -> Mux1/2
  Demux/5 -> D Flip-Flop4/1
  D Flip-Flop1/1 -> Mux/2
  D Flip-Flop2/1 -> Mux/3
  D Flip-Flop5/1 -> Mux/6
  Demux/6 -> D Flip-Flop5/1
  In3/1 -> D Flip-Flop7/3, D Flip-Flop6/3, D Flip-Flop5/3, D Flip-Flop4/3, D Flip-Flop3/3, D Flip-Flop2/3, D Flip-Flop1/3, D Flip-Flop/3
  Demux/7 -> D Flip-Flop6/1
  D Flip-Flop6/1 -> Mux/7
  Demux/3 -> D Flip-Flop2/1
  Mux/1 -> Out1/1
  In2/1 -> D Flip-Flop7/2, D Flip-Flop6/2, D Flip-Flop5/2, D Flip-Flop4/2, D Flip-Flop3/2, D Flip-Flop2/2, D Flip-Flop/2, D Flip-Flop1/2
  Demux/2 -> D Flip-Flop1/1
  Demux/8 -> D Flip-Flop7/1
  D Flip-Flop5/2 -> Mux1/6
  D Flip-Flop4/1 -> Mux/5
  D Flip-Flop7/2 -> Mux1/8
  D Flip-Flop7/1 -> Mux/8
  Demux/4 -> D Flip-Flop3/1
  Mux1/1 -> Display/1
  D Flip-Flop2/2 -> Mux1/3
  In1/1 -> Demux/1
  D Flip-Flop4/2 -> Mux1/5
  Demux/1 -> D Flip-Flop/1
  D Flip-Flop/2 -> Mux1/1
  D Flip-Flop3/1 -> Mux/4
  D Flip-Flop/1 -> Mux/1
  D Flip-Flop3/2 -> Mux1/4

== system cpu_von_nuemann/CPU/MU/Multiplier H bit/Subsystem2 ==
  In1 : Inport
  In2 : Inport  Port=2
  In3 : Inport  Port=3
  D Flip-Flop{,1..7} (8 alike) : simulink_extras/Flip Flops/D Flip-Flop
  Demux : Demux  Outputs=8
  Display : Display
  Mux : Mux  Inputs=8
  Mux1 : Mux  Inputs=8
  Out1 : Outport
  wires:
  D Flip-Flop6/2 -> Mux1/7
  D Flip-Flop1/2 -> Mux1/2
  Demux/5 -> D Flip-Flop4/1
  D Flip-Flop1/1 -> Mux/2
  D Flip-Flop2/1 -> Mux/3
  D Flip-Flop5/1 -> Mux/6
  Demux/6 -> D Flip-Flop5/1
  In3/1 -> D Flip-Flop7/3, D Flip-Flop6/3, D Flip-Flop5/3, D Flip-Flop4/3, D Flip-Flop3/3, D Flip-Flop2/3, D Flip-Flop1/3, D Flip-Flop/3
  Demux/7 -> D Flip-Flop6/1
  D Flip-Flop6/1 -> Mux/7
  Demux/3 -> D Flip-Flop2/1
  Mux/1 -> Out1/1
  In2/1 -> D Flip-Flop7/2, D Flip-Flop6/2, D Flip-Flop5/2, D Flip-Flop4/2, D Flip-Flop3/2, D Flip-Flop2/2, D Flip-Flop/2, D Flip-Flop1/2
  Demux/2 -> D Flip-Flop1/1
  Demux/8 -> D Flip-Flop7/1
  D Flip-Flop5/2 -> Mux1/6
  D Flip-Flop4/1 -> Mux/5
  D Flip-Flop7/2 -> Mux1/8
  D Flip-Flop7/1 -> Mux/8
  Demux/4 -> D Flip-Flop3/1
  Mux1/1 -> Display/1
  D Flip-Flop2/2 -> Mux1/3
  In1/1 -> Demux/1
  D Flip-Flop4/2 -> Mux1/5
  Demux/1 -> D Flip-Flop/1
  D Flip-Flop/2 -> Mux1/1
  D Flip-Flop3/1 -> Mux/4
  D Flip-Flop/1 -> Mux/1
  D Flip-Flop3/2 -> Mux1/4

== system cpu_von_nuemann/CPU/MU/Multiplier H bit/Subsystem3 ==
  In1 : Inport
  In2 : Inport  Port=2
  In3 : Inport  Port=3
  D Flip-Flop{,1..7} (8 alike) : simulink_extras/Flip Flops/D Flip-Flop
  Demux : Demux  Outputs=8
  Display : Display
  Mux : Mux  Inputs=8
  Mux1 : Mux  Inputs=8
  Out1 : Outport
  wires:
  D Flip-Flop6/2 -> Mux1/7
  D Flip-Flop1/2 -> Mux1/2
  Demux/5 -> D Flip-Flop4/1
  D Flip-Flop1/1 -> Mux/2
  D Flip-Flop2/1 -> Mux/3
  D Flip-Flop5/1 -> Mux/6
  Demux/6 -> D Flip-Flop5/1
  In3/1 -> D Flip-Flop7/3, D Flip-Flop6/3, D Flip-Flop5/3, D Flip-Flop4/3, D Flip-Flop3/3, D Flip-Flop2/3, D Flip-Flop1/3, D Flip-Flop/3
  Demux/7 -> D Flip-Flop6/1
  D Flip-Flop6/1 -> Mux/7
  Demux/3 -> D Flip-Flop2/1
  Mux/1 -> Out1/1
  In2/1 -> D Flip-Flop7/2, D Flip-Flop6/2, D Flip-Flop5/2, D Flip-Flop4/2, D Flip-Flop3/2, D Flip-Flop2/2, D Flip-Flop/2, D Flip-Flop1/2
  Demux/2 -> D Flip-Flop1/1
  Demux/8 -> D Flip-Flop7/1
  D Flip-Flop5/2 -> Mux1/6
  D Flip-Flop4/1 -> Mux/5
  D Flip-Flop7/2 -> Mux1/8
  D Flip-Flop7/1 -> Mux/8
  Demux/4 -> D Flip-Flop3/1
  Mux1/1 -> Display/1
  D Flip-Flop2/2 -> Mux1/3
  In1/1 -> Demux/1
  D Flip-Flop4/2 -> Mux1/5
  Demux/1 -> D Flip-Flop/1
  D Flip-Flop/2 -> Mux1/1
  D Flip-Flop3/1 -> Mux/4
  D Flip-Flop/1 -> Mux/1
  D Flip-Flop3/2 -> Mux1/4

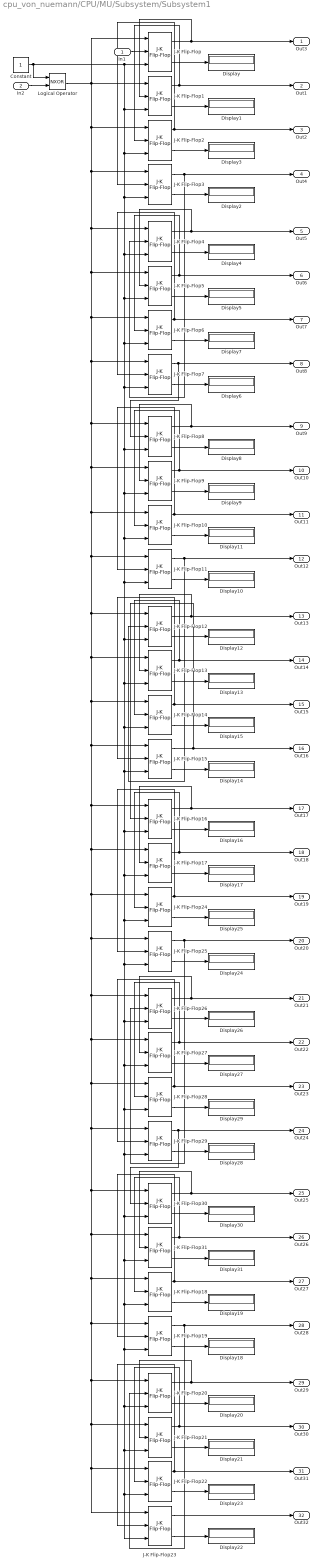
== system cpu_von_nuemann/CPU/MU/Subsystem/Subsystem1 ==
  In1 : Inport
  In2 : Inport  Port=2
  Constant : Constant  OutDataTypeStr=boolean
  Display{,1..31} (32 alike) : Display
  J-K Flip-Flop{,1..31} (32 alike) : simulink_extras/Flip Flops/J-K Flip-Flop  initial_condition=0
  Logical Operator : Logic  Operator=NXOR  AllPortsSameDT=off  OutDataTypeStr=boolean
  Out3 : Outport
  Out1 : Outport  Port=2
  Out2 : Outport  Port=3
  Out4 : Outport  Port=4
  Out5 : Outport  Port=5
  Out6 : Outport  Port=6
  Out7 : Outport  Port=7
  Out8 : Outport  Port=8
  Out9 : Outport  Port=9
  Out10 : Outport  Port=10
  Out11 : Outport  Port=11
  Out12 : Outport  Port=12
  Out13 : Outport  Port=13
  Out14 : Outport  Port=14
  Out15 : Outport  Port=15
  Out16 : Outport  Port=16
  Out17 : Outport  Port=17
  Out18 : Outport  Port=18
  Out19 : Outport  Port=19
  Out20 : Outport  Port=20
  Out21 : Outport  Port=21
  Out22 : Outport  Port=22
  Out23 : Outport  Port=23
  Out24 : Outport  Port=24
  Out25 : Outport  Port=25
  Out26 : Outport  Port=26
  Out27 : Outport  Port=27
  Out28 : Outport  Port=28
  Out29 : Outport  Port=29
  Out30 : Outport  Port=30
  Out31 : Outport  Port=31
  Out32 : Outport  Port=32
  wires:
  J-K Flip-Flop23/1 -> Out32/1
  J-K Flip-Flop7/2 -> Display6/1
  J-K Flip-Flop4/2 -> Display4/1
  J-K Flip-Flop/2 -> Display/1
  J-K Flip-Flop25/2 -> Display24/1
  J-K Flip-Flop1/2 -> Display1/1
  J-K Flip-Flop/1 -> Out3/1, J-K Flip-Flop1/2
  J-K Flip-Flop20/2 -> Display20/1
  J-K Flip-Flop27/1 -> Out22/1, J-K Flip-Flop28/2
  J-K Flip-Flop26/2 -> Display26/1
  J-K Flip-Flop21/1 -> Out30/1, J-K Flip-Flop22/2
  J-K Flip-Flop19/1 -> Out28/1, J-K Flip-Flop20/2
  J-K Flip-Flop12/2 -> Display12/1
  J-K Flip-Flop26/1 -> Out21/1, J-K Flip-Flop27/2
  J-K Flip-Flop1/1 -> Out1/1, J-K Flip-Flop2/2
  J-K Flip-Flop31/1 -> Out26/1, J-K Flip-Flop18/2
  J-K Flip-Flop13/1 -> Out14/1, J-K Flip-Flop14/2
  J-K Flip-Flop22/1 -> Out31/1, J-K Flip-Flop23/2
  J-K Flip-Flop9/2 -> Display9/1
  J-K Flip-Flop14/1 -> Out15/1, J-K Flip-Flop15/2
  J-K Flip-Flop22/2 -> Display23/1
  J-K Flip-Flop30/1 -> Out25/1, J-K Flip-Flop31/2
  J-K Flip-Flop11/2 -> Display10/1
  J-K Flip-Flop28/2 -> Display29/1
  J-K Flip-Flop20/1 -> Out29/1, J-K Flip-Flop21/2
  J-K Flip-Flop17/1 -> Out18/1, J-K Flip-Flop24/2
  J-K Flip-Flop19/2 -> Display18/1
  J-K Flip-Flop15/2 -> Display14/1
  J-K Flip-Flop27/2 -> Display27/1
  J-K Flip-Flop9/1 -> Out10/1, J-K Flip-Flop10/2
  J-K Flip-Flop29/1 -> Out24/1, J-K Flip-Flop30/2
  J-K Flip-Flop8/2 -> Display8/1
  J-K Flip-Flop31/2 -> Display31/1
  J-K Flip-Flop11/1 -> Out12/1, J-K Flip-Flop12/2
  J-K Flip-Flop5/1 -> Out6/1, J-K Flip-Flop6/2
  J-K Flip-Flop3/1 -> Out4/1, J-K Flip-Flop4/2
  J-K Flip-Flop18/2 -> Display19/1
  J-K Flip-Flop3/2 -> Display2/1
  J-K Flip-Flop16/2 -> Display16/1
  J-K Flip-Flop17/2 -> Display17/1
  J-K Flip-Flop18/1 -> Out27/1, J-K Flip-Flop19/2
  J-K Flip-Flop25/1 -> Out20/1, J-K Flip-Flop26/2
  J-K Flip-Flop6/1 -> Out7/1, J-K Flip-Flop7/2
  J-K Flip-Flop16/1 -> Out17/1, J-K Flip-Flop17/2
  In1/1 -> J-K Flip-Flop/2
  J-K Flip-Flop24/1 -> Out19/1, J-K Flip-Flop25/2
  J-K Flip-Flop5/2 -> Display5/1
  J-K Flip-Flop24/2 -> Display25/1
  J-K Flip-Flop12/1 -> Out13/1, J-K Flip-Flop13/2
  J-K Flip-Flop29/2 -> Display28/1
  J-K Flip-Flop23/2 -> Display22/1
  J-K Flip-Flop13/2 -> Display13/1
  J-K Flip-Flop28/1 -> Out23/1, J-K Flip-Flop29/2
  J-K Flip-Flop7/1 -> Out8/1, J-K Flip-Flop8/2
  J-K Flip-Flop8/1 -> Out9/1, J-K Flip-Flop9/2
  J-K Flip-Flop4/1 -> Out5/1, J-K Flip-Flop5/2
  J-K Flip-Flop30/2 -> Display30/1
  J-K Flip-Flop2/2 -> Display3/1
  J-K Flip-Flop10/1 -> Out11/1, J-K Flip-Flop11/2
  J-K Flip-Flop14/2 -> Display15/1
  J-K Flip-Flop10/2 -> Display11/1
  J-K Flip-Flop2/1 -> Out2/1, J-K Flip-Flop3/2
  J-K Flip-Flop6/2 -> Display7/1
  J-K Flip-Flop21/2 -> Display21/1
  J-K Flip-Flop15/1 -> Out16/1, J-K Flip-Flop16/2
  Constant/1 -> Logical Operator/1, J-K Flip-Flop23/3, J-K Flip-Flop22/3, J-K Flip-Flop21/3, J-K Flip-Flop20/3, J-K Flip-Flop19/3, J-K Flip-Flop18/3, J-K Flip-Flop31/3, J-K Flip-Flop30/3, J-K Flip-Flop29/3, J-K Flip-Flop28/3, J-K Flip-Flop27/3, J-K Flip-Flop26/3, J-K Flip-Flop25/3, J-K Flip-Flop24/3, J-K Flip-Flop17/3, J-K Flip-Flop16/3, J-K Flip-Flop15/3, J-K Flip-Flop14/3, J-K Flip-Flop13/3, J-K Flip-Flop12/3, J-K Flip-Flop11/3, J-K Flip-Flop10/3, J-K Flip-Flop9/3, J-K Flip-Flop8/3, J-K Flip-Flop7/3, J-K Flip-Flop6/3, J-K Flip-Flop5/3, J-K Flip-Flop4/3, J-K Flip-Flop3/3, J-K Flip-Flop2/3, J-K Flip-Flop1/3, J-K Flip-Flop/3
  In2/1 -> Logical Operator/2
  Logical Operator/1 -> J-K Flip-Flop23/1, J-K Flip-Flop22/1, J-K Flip-Flop21/1, J-K Flip-Flop20/1, J-K Flip-Flop19/1, J-K Flip-Flop18/1, J-K Flip-Flop31/1, J-K Flip-Flop30/1, J-K Flip-Flop29/1, J-K Flip-Flop28/1, J-K Flip-Flop27/1, J-K Flip-Flop26/1, J-K Flip-Flop25/1, J-K Flip-Flop24/1, J-K Flip-Flop17/1, J-K Flip-Flop16/1, J-K Flip-Flop15/1, J-K Flip-Flop14/1, J-K Flip-Flop13/1, J-K Flip-Flop12/1, J-K Flip-Flop11/1, J-K Flip-Flop10/1, J-K Flip-Flop9/1, J-K Flip-Flop8/1, J-K Flip-Flop7/1, J-K Flip-Flop6/1, J-K Flip-Flop5/1, J-K Flip-Flop4/1, J-K Flip-Flop3/1, J-K Flip-Flop2/1, J-K Flip-Flop1/1, J-K Flip-Flop/1

== system cpu_von_nuemann/CPU/MU/reg A/Subsystem ==
  In1 : Inport
  In2 : Inport  Port=2
  In3 : Inport  Port=3
  D Flip-Flop{,1..7} (8 alike) : simulink_extras/Flip Flops/D Flip-Flop
  Demux : Demux  Outputs=8
  Display : Display
  Mux : Mux  Inputs=8
  Mux1 : Mux  Inputs=8
  Out1 : Outport
  wires:
  D Flip-Flop6/2 -> Mux1/7
  D Flip-Flop1/2 -> Mux1/2
  Demux/5 -> D Flip-Flop4/1
  D Flip-Flop1/1 -> Mux/2
  D Flip-Flop2/1 -> Mux/3
  D Flip-Flop5/1 -> Mux/6
  Demux/6 -> D Flip-Flop5/1
  In3/1 -> D Flip-Flop7/3, D Flip-Flop6/3, D Flip-Flop5/3, D Flip-Flop4/3, D Flip-Flop3/3, D Flip-Flop2/3, D Flip-Flop1/3, D Flip-Flop/3
  Demux/7 -> D Flip-Flop6/1
  D Flip-Flop6/1 -> Mux/7
  Demux/3 -> D Flip-Flop2/1
  Mux/1 -> Out1/1
  In2/1 -> D Flip-Flop7/2, D Flip-Flop6/2, D Flip-Flop5/2, D Flip-Flop4/2, D Flip-Flop3/2, D Flip-Flop2/2, D Flip-Flop/2, D Flip-Flop1/2
  Demux/2 -> D Flip-Flop1/1
  Demux/8 -> D Flip-Flop7/1
  D Flip-Flop5/2 -> Mux1/6
  D Flip-Flop4/1 -> Mux/5
  D Flip-Flop7/2 -> Mux1/8
  D Flip-Flop7/1 -> Mux/8
  Demux/4 -> D Flip-Flop3/1
  Mux1/1 -> Display/1
  D Flip-Flop2/2 -> Mux1/3
  In1/1 -> Demux/1
  D Flip-Flop4/2 -> Mux1/5
  Demux/1 -> D Flip-Flop/1
  D Flip-Flop/2 -> Mux1/1
  D Flip-Flop3/1 -> Mux/4
  D Flip-Flop/1 -> Mux/1
  D Flip-Flop3/2 -> Mux1/4

== system cpu_von_nuemann/CPU/MU/reg A/Subsystem1 ==
  In1 : Inport
  In2 : Inport  Port=2
  In3 : Inport  Port=3
  D Flip-Flop{,1..7} (8 alike) : simulink_extras/Flip Flops/D Flip-Flop
  Demux : Demux  Outputs=8
  Display : Display
  Mux : Mux  Inputs=8
  Mux1 : Mux  Inputs=8
  Out1 : Outport
  wires:
  D Flip-Flop6/2 -> Mux1/7
  D Flip-Flop1/2 -> Mux1/2
  Demux/5 -> D Flip-Flop4/1
  D Flip-Flop1/1 -> Mux/2
  D Flip-Flop2/1 -> Mux/3
  D Flip-Flop5/1 -> Mux/6
  Demux/6 -> D Flip-Flop5/1
  In3/1 -> D Flip-Flop7/3, D Flip-Flop6/3, D Flip-Flop5/3, D Flip-Flop4/3, D Flip-Flop3/3, D Flip-Flop2/3, D Flip-Flop1/3, D Flip-Flop/3
  Demux/7 -> D Flip-Flop6/1
  D Flip-Flop6/1 -> Mux/7
  Demux/3 -> D Flip-Flop2/1
  Mux/1 -> Out1/1
  In2/1 -> D Flip-Flop7/2, D Flip-Flop6/2, D Flip-Flop5/2, D Flip-Flop4/2, D Flip-Flop3/2, D Flip-Flop2/2, D Flip-Flop/2, D Flip-Flop1/2
  Demux/2 -> D Flip-Flop1/1
  Demux/8 -> D Flip-Flop7/1
  D Flip-Flop5/2 -> Mux1/6
  D Flip-Flop4/1 -> Mux/5
  D Flip-Flop7/2 -> Mux1/8
  D Flip-Flop7/1 -> Mux/8
  Demux/4 -> D Flip-Flop3/1
  Mux1/1 -> Display/1
  D Flip-Flop2/2 -> Mux1/3
  In1/1 -> Demux/1
  D Flip-Flop4/2 -> Mux1/5
  Demux/1 -> D Flip-Flop/1
  D Flip-Flop/2 -> Mux1/1
  D Flip-Flop3/1 -> Mux/4
  D Flip-Flop/1 -> Mux/1
  D Flip-Flop3/2 -> Mux1/4

== system cpu_von_nuemann/CPU/MU/reg A/Subsystem2 ==
  In1 : Inport
  In2 : Inport  Port=2
  In3 : Inport  Port=3
  D Flip-Flop{,1..7} (8 alike) : simulink_extras/Flip Flops/D Flip-Flop
  Demux : Demux  Outputs=8
  Display : Display
  Mux : Mux  Inputs=8
  Mux1 : Mux  Inputs=8
  Out1 : Outport
  wires:
  D Flip-Flop6/2 -> Mux1/7
  D Flip-Flop1/2 -> Mux1/2
  Demux/5 -> D Flip-Flop4/1
  D Flip-Flop1/1 -> Mux/2
  D Flip-Flop2/1 -> Mux/3
  D Flip-Flop5/1 -> Mux/6
  Demux/6 -> D Flip-Flop5/1
  In3/1 -> D Flip-Flop7/3, D Flip-Flop6/3, D Flip-Flop5/3, D Flip-Flop4/3, D Flip-Flop3/3, D Flip-Flop2/3, D Flip-Flop1/3, D Flip-Flop/3
  Demux/7 -> D Flip-Flop6/1
  D Flip-Flop6/1 -> Mux/7
  Demux/3 -> D Flip-Flop2/1
  Mux/1 -> Out1/1
  In2/1 -> D Flip-Flop7/2, D Flip-Flop6/2, D Flip-Flop5/2, D Flip-Flop4/2, D Flip-Flop3/2, D Flip-Flop2/2, D Flip-Flop/2, D Flip-Flop1/2
  Demux/2 -> D Flip-Flop1/1
  Demux/8 -> D Flip-Flop7/1
  D Flip-Flop5/2 -> Mux1/6
  D Flip-Flop4/1 -> Mux/5
  D Flip-Flop7/2 -> Mux1/8
  D Flip-Flop7/1 -> Mux/8
  Demux/4 -> D Flip-Flop3/1
  Mux1/1 -> Display/1
  D Flip-Flop2/2 -> Mux1/3
  In1/1 -> Demux/1
  D Flip-Flop4/2 -> Mux1/5
  Demux/1 -> D Flip-Flop/1
  D Flip-Flop/2 -> Mux1/1
  D Flip-Flop3/1 -> Mux/4
  D Flip-Flop/1 -> Mux/1
  D Flip-Flop3/2 -> Mux1/4

== system cpu_von_nuemann/CPU/MU/reg A/Subsystem3 ==
  In1 : Inport
  In2 : Inport  Port=2
  In3 : Inport  Port=3
  D Flip-Flop{,1..7} (8 alike) : simulink_extras/Flip Flops/D Flip-Flop
  Demux : Demux  Outputs=8
  Display : Display
  Mux : Mux  Inputs=8
  Mux1 : Mux  Inputs=8
  Out1 : Outport
  wires:
  D Flip-Flop6/2 -> Mux1/7
  D Flip-Flop1/2 -> Mux1/2
  Demux/5 -> D Flip-Flop4/1
  D Flip-Flop1/1 -> Mux/2
  D Flip-Flop2/1 -> Mux/3
  D Flip-Flop5/1 -> Mux/6
  Demux/6 -> D Flip-Flop5/1
  In3/1 -> D Flip-Flop7/3, D Flip-Flop6/3, D Flip-Flop5/3, D Flip-Flop4/3, D Flip-Flop3/3, D Flip-Flop2/3, D Flip-Flop1/3, D Flip-Flop/3
  Demux/7 -> D Flip-Flop6/1
  D Flip-Flop6/1 -> Mux/7
  Demux/3 -> D Flip-Flop2/1
  Mux/1 -> Out1/1
  In2/1 -> D Flip-Flop7/2, D Flip-Flop6/2, D Flip-Flop5/2, D Flip-Flop4/2, D Flip-Flop3/2, D Flip-Flop2/2, D Flip-Flop/2, D Flip-Flop1/2
  Demux/2 -> D Flip-Flop1/1
  Demux/8 -> D Flip-Flop7/1
  D Flip-Flop5/2 -> Mux1/6
  D Flip-Flop4/1 -> Mux/5
  D Flip-Flop7/2 -> Mux1/8
  D Flip-Flop7/1 -> Mux/8
  Demux/4 -> D Flip-Flop3/1
  Mux1/1 -> Display/1
  D Flip-Flop2/2 -> Mux1/3
  In1/1 -> Demux/1
  D Flip-Flop4/2 -> Mux1/5
  Demux/1 -> D Flip-Flop/1
  D Flip-Flop/2 -> Mux1/1
  D Flip-Flop3/1 -> Mux/4
  D Flip-Flop/1 -> Mux/1
  D Flip-Flop3/2 -> Mux1/4

== system cpu_von_nuemann/CPU/MU/reg AH/Subsystem ==
  In1 : Inport
  In2 : Inport  Port=2
  In3 : Inport  Port=3
  D Flip-Flop{,1..7} (8 alike) : simulink_extras/Flip Flops/D Flip-Flop
  Demux : Demux  Outputs=8
  Display : Display
  Mux : Mux  Inputs=8
  Mux1 : Mux  Inputs=8
  Out1 : Outport
  wires:
  D Flip-Flop6/2 -> Mux1/7
  D Flip-Flop1/2 -> Mux1/2
  Demux/5 -> D Flip-Flop4/1
  D Flip-Flop1/1 -> Mux/2
  D Flip-Flop2/1 -> Mux/3
  D Flip-Flop5/1 -> Mux/6
  Demux/6 -> D Flip-Flop5/1
  In3/1 -> D Flip-Flop7/3, D Flip-Flop6/3, D Flip-Flop5/3, D Flip-Flop4/3, D Flip-Flop3/3, D Flip-Flop2/3, D Flip-Flop1/3, D Flip-Flop/3
  Demux/7 -> D Flip-Flop6/1
  D Flip-Flop6/1 -> Mux/7
  Demux/3 -> D Flip-Flop2/1
  Mux/1 -> Out1/1
  In2/1 -> D Flip-Flop7/2, D Flip-Flop6/2, D Flip-Flop5/2, D Flip-Flop4/2, D Flip-Flop3/2, D Flip-Flop2/2, D Flip-Flop/2, D Flip-Flop1/2
  Demux/2 -> D Flip-Flop1/1
  Demux/8 -> D Flip-Flop7/1
  D Flip-Flop5/2 -> Mux1/6
  D Flip-Flop4/1 -> Mux/5
  D Flip-Flop7/2 -> Mux1/8
  D Flip-Flop7/1 -> Mux/8
  Demux/4 -> D Flip-Flop3/1
  Mux1/1 -> Display/1
  D Flip-Flop2/2 -> Mux1/3
  In1/1 -> Demux/1
  D Flip-Flop4/2 -> Mux1/5
  Demux/1 -> D Flip-Flop/1
  D Flip-Flop/2 -> Mux1/1
  D Flip-Flop3/1 -> Mux/4
  D Flip-Flop/1 -> Mux/1
  D Flip-Flop3/2 -> Mux1/4
